simulink model "VehicleWithFourSpeedTransmission"  (R2025b)
settings: Solver=VariableStepAuto  StartTime=0.0  StopTime=50  FixedStep=1e-3  RelTol=1e-3  AbsTol=1e-3  EnableMultiTasking=on
model workspace (MAT data in the model file):
  DOWN_TABLE = [0  5  20  35; 0  5  20  35; 0  5  25  40; 0  5  30  50; 0  30  50  80; 0  30  50  80]
  DOWN_TH_BP = [0; 0.05; 0.4; 0.5; 0.9; 1]
  TWAIT = 2
  UP_TABLE = [10  30  50  1000000; 10  30  50  1000000; 15  30  50  1000000; 23  41  60  1000000; 40  70  100  1000000; 40  70  100  1000000]
  UP_TH_BP = [0; 0.25; 0.35; 0.5; 0.9; 1]
  clutchRise = 0.1
  eff_tor_rad = 0.4
  engagement_area = 0.0025
  fric_coeff = 0.5
  num_fric_surf = 6
  p0 = 2000000
  peak_normal = 0.55
  pressThresh = 0.05
  velTol = 0.001
libraries: sdl_lib x13, nesl_utility x12, fl_lib x11
CloseFcn:
  | try,close(h1_VehicleWithFourSpeedTransmission),end
  | clear h1_VehicleWithFourSpeedTransmission
  | 
  | clear simlog_VehicleWithFourSpeedTransmission
  | clear logsout_VehicleWithFourSpeedTransmission
Description:
  | Vehicle with Four-Speed Transmission
settings Model: FPTRunName=Active  ExtModeAutoUpdateStatusClock=off  Creator=The MathWorks, Inc.  LastModifiedBy=mateu
settings SolverCC: AutoScaleAbsTol=off  ZcThreshold=0  AlgebraicLoopSolver=TrustRegion
settings DataIOCC: LimitDataPoints=on  MaxDataPoints=10000  SaveOutput=off  DSMLogging=off  SaveTime=off  ReturnWorkspaceOutputs=off  SignalLoggingName=logsout_VehicleWithFourSpeedTransmission
settings OptimizationCC: ExpressionDepthLimit=2147483647.0  InitFltsAndDblsToZero=on  LifeSpan=inf
settings DebuggingCC: AlgebraicLoopMsg=none  SaveWithParameterizedLinksMsg=none  MergeDetectMultiDrivingBlocksExec=none  CheckExecutionContextPreStartOutputMsg=on  SignalResolutionControl=TryResolveAllWithWarning  MaskedZcDiagnostic=none  MultiTaskDSMMsg=warning  MultiTaskCondExecSysMsg=none  SigSpecEnsureSampleTimeMsg=none  UnconnectedInputMsg=warning  UnconnectedOutputMsg=warning  UnconnectedLineMsg=warning  AllowSymbolicDim=off  StateNameClashWarn=warning  PregeneratedLibrarySubsystemCodeDiagnostic=none  SFUnexpectedBacktrackingDiag=warning  SFNoUnconditionalDefaultTransitionDiag=warning  SFExecutionAtInitializationDiag=none  ArithmeticOperatorsInVariantConditions=warning
settings HardwareCC: ProdBitPerPointer=32.0  ProdBitPerSizeT=32.0  ProdBitPerPtrDiffT=32.0  ProdLargestAtomicFloat=None  ProdIntDivRoundTo=Undefined  ProdEndianess=Unspecified  ProdWordSize=32.0  ProdHWDeviceType=32-bit Generic  TargetBitPerPointer=64.0  TargetBitPerSizeT=64.0  TargetBitPerPtrDiffT=64.0  TargetLongLongMode=on  TargetIntDivRoundTo=Zero  TargetEndianess=LittleEndian  TargetWordSize=64.0  TargetHWDeviceType=MATLAB Host  ProdEqTarget=off
settings ModelReferenceCC: UpdateModelReferenceTargets=IfOutOfDate  EnableRefExpFcnMdlSchedulingChecks=on  PropagateSignalLabelsOutOfModel=off
settings SFSimCC: SimUseLocalCustomCode=off
settings RTWCC: RTWUseLocalCustomCode=off  GPUComputeCapability=3.5  DLArmComputeVersion=19.05
settings CodeAppCC: StateflowObjectComments=on
settings GRTTargetCC: TargetLangStandard=C89/C90 (ANSI)  CombineOutputUpdateFcns=off  GRTInterface=on
settings ConfigComp: CovScope=ReferencedModels  CovIncludeTopModel=off  CovMetricSettings=dw  CovSaveCumulativeToWorkspaceVar=on  CovSaveSingleToWorkspaceVar=on  CovExternalEMLEnable=off
settings SimscapeCC: SimscapeLogName=simlog_VehicleWithFourSpeedTransmission  SimscapeLogDataHistory=15000.0

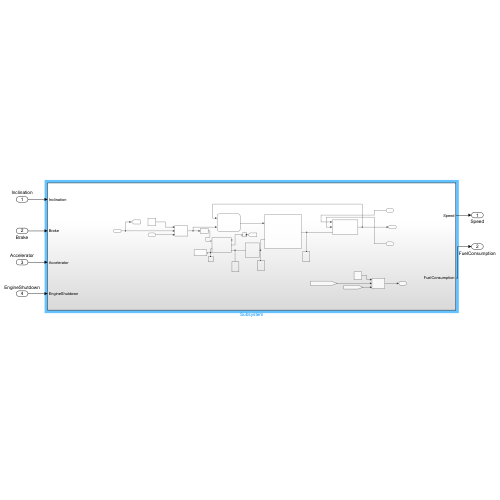
[thumbnail: Simulink's stored preview of the top-level diagram]
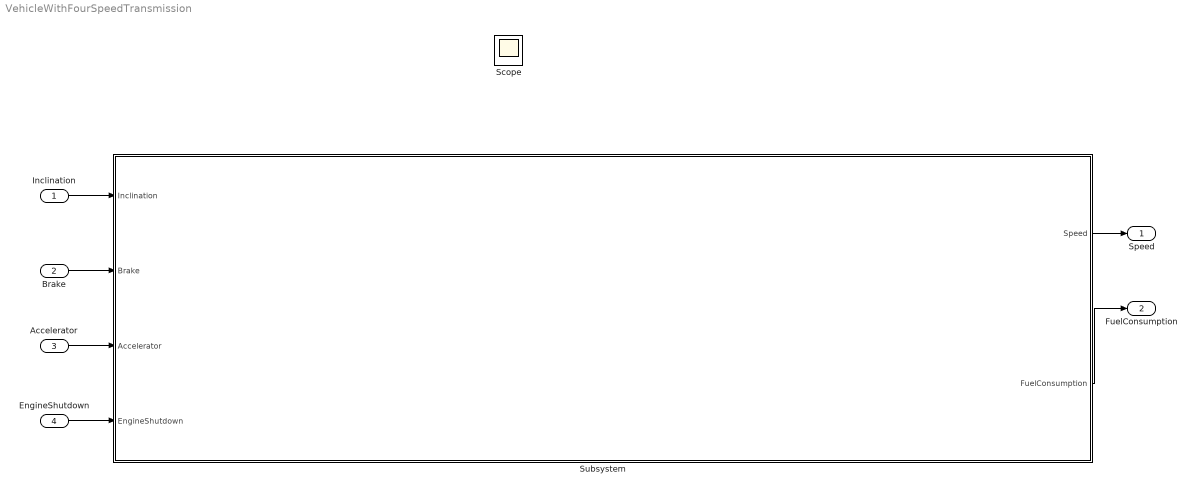
== system VehicleWithFourSpeedTransmission ==
  Inclination : Inport
  Brake : Inport  Port=2
  Accelerator : Inport  Port=3
  EngineShutdown : Inport  Port=4
  Subsystem : Subsystem
  Speed : Outport
  FuelConsumption : Outport  Port=2
  Scope : Scope
      settings: ActiveDisplayYMinimum=0.625  ActiveDisplayYMaximum=4.375
  wires:
  Inclination/1 -> Subsystem/1(Inclination)
  Brake/1 -> Subsystem/2(Brake)
  Accelerator/1 -> Subsystem/3(Accelerator)
  Subsystem/1(Speed) -> Speed/1
  Subsystem/2(FuelConsumption) -> FuelConsumption/1
  EngineShutdown/1 -> Subsystem/4(EngineShutdown)

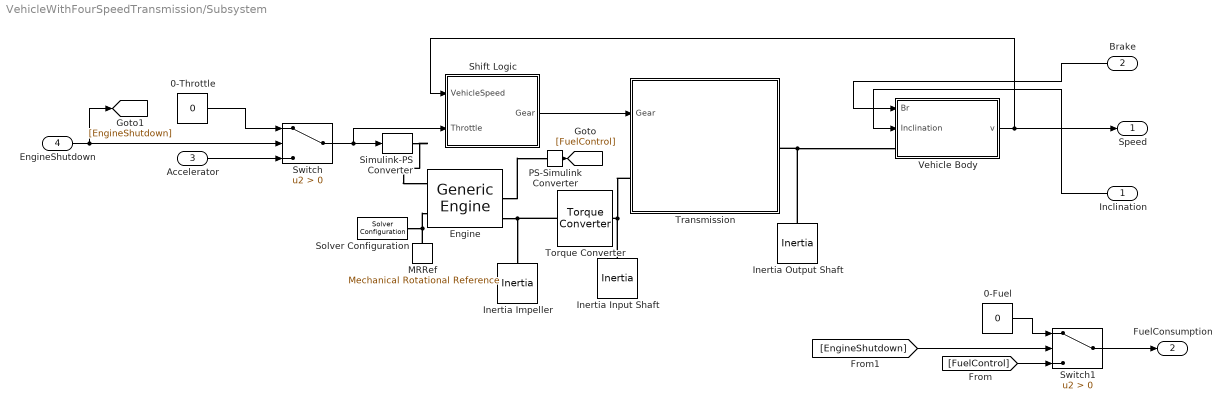
== system VehicleWithFourSpeedTransmission/Subsystem ==
  Inclination : Inport
  Brake : Inport  Port=2
  Accelerator : Inport  Port=3
  EngineShutdown : Inport  Port=4
  0-Fuel : Constant  Value=0
  0-Throttle : Constant  Value=0
  Engine : sdl_lib/Engines & Motors/Generic Engine  input_type=sdl.enum.GenericEngineInputType.NormalizedThrottle  model_parameterization=1  engine_type=1  Trq_max=380 N*m  w_Trq_max=4300 rpm  P_max=1.5e+5 W  w_P_max=4.5e+3 rpm  w_max=6e+3 rpm  w_min=500 rpm  w_tab=[ 500 1000 2e+3 3e+3 4e+3 5e+3 6e+3 7e+3 ] rpm  trq_tab=[ 380 380 380 380 350 280 200 80 ] N*m  pwr_tab=[ 2e+4 4e+4 7.8e+4 1.2e+5 1.45e+5 1.48e+5 1.25e+5 6e+4 ] W  interp_method=simscape.enum.interpolation.linear  w_thr=100 rpm  model_inertia=1  inertia=0.08 kg*m^2  initial_velocity=960 rpm  model_time_constant=1  time_constant=0.4 s  initial_normalized_throttle=0  fc_model=sdl.enum.fuel_consumption_model.FuelSpeedTorque  fc_per_rev=25 mg/rev  fc_w_tab=[ 1000 2e+3 3e+3 4e+3 5e+3 6e+3 ] rpm  fc_trq_tab=[ 0 80 160 200 240 320 360 400 ] N*m  fc_tab=[ 0.5 0.9 1.4 1.6 1.9 2.7 3.4 4.4; 1 1.7 2.7 3.1 3.6 5 6 7.4; 1.4 2.7 4 4.8 5.6 7.5 8.5 10.5; 2 3.6 5.8 6.7 8 10.4 11.7 13.3; 2.5 4.8 7.9 9.4 10.8 14 16.2 18.6; 3.1 6 10.3 11.9 13.8 18.4 22 26.5 ] g/s  bmep_tab=[ 0 250 500 625 750 1000 1.15e+3 1.25e+3 ] kPa  bsfc_tab=[ 410 380 300 280 270 290 320 380; 410 370 290 270 260 270 285 320; 415 380 290 275 265 270 270 300; 420 390 310 290 285 280 280 285; 430 410 340 320 310 300 310 320; 450 430 370 340 330 330 350 380 ] g/hr/kW  fc_interp_method=simscape.enum.interpolation.linear  displaced_volume=400 cm^3  rev_per_cycle=2  idle_speed=true  idle_speed_reference=1000 rpm  tau_controller=1 s  idle_w_thr=1 rpm  redline=0  redline_speed=5000 rpm  tau_redline=1 s  redline_w_thr=1 rpm
      settings: InternalSimscapePortConfiguration="{\"Bottom\":[],\"Left\":[{\"id\":\"ThrNorm\",\"label\":\"Thr\",\"type\":\"input\"},{\"id\":\"B\",\"label\":\"B\",\"type\":\"foundation.mechanical.rotational.rotational\"}],\"Right\":[{\"id\":\"P\",\"label\":\"P\",\"type\":\"output\"},{\"id\":\"FC\",\"label\":\"FC\",\"type\":\"output\"},{\"id\":\"F\",\"label\":\"F\",\"type\":\"foundation.mechanical.rotational.rotational\"}],\"Top\":[]}"
  Inertia Impeller : fl_lib/Mechanical/Rotational Elements/Inertia  inertia=0.02 kg*m^2  num_ports=foundation.enum.numPorts2.one  w_specify=on  w_priority=None  w=0 rpm  w_nominal_specify=off  w_nominal_value=1  w_nominal_unit=rad/s  t_specify=off  t_priority=High  t=0 N*m  t_nominal_specify=off  t_nominal_value=1  t_nominal_unit=N*m
  Inertia Input Shaft : fl_lib/Mechanical/Rotational Elements/Inertia  inertia=1e-2 kg*m^2  num_ports=foundation.enum.numPorts2.one  w_specify=on  w_priority=High  w=0 rad/s  w_nominal_specify=off  w_nominal_value=1  w_nominal_unit=rad/s  t_specify=off  t_priority=High  t=0 N*m  t_nominal_specify=off  t_nominal_value=1  t_nominal_unit=N*m
  Inertia Output Shaft : fl_lib/Mechanical/Rotational Elements/Inertia  inertia=1e-1 kg*m^2  num_ports=foundation.enum.numPorts2.one  w_specify=on  w_priority=None  w=0 rad/s  w_nominal_specify=off  w_nominal_value=1  w_nominal_unit=rad/s  t_specify=off  t_priority=High  t=0 N*m  t_nominal_specify=off  t_nominal_value=1  t_nominal_unit=N*m
  MRRef : fl_lib/Mechanical/Rotational Elements/Mechanical Rotational Reference
  PS-Simulink Converter : nesl_utility/PS-Simulink Converter  PhysicalDomain=network_engine_domain  SubClassName=ps_output  LeftPortType=input  RightPortType=output  PseudoPeriodic=off  Frequencies=[]  VectorFormat=inherit  Unit=inherit  AffineConversion=off
  Shift Logic : Stateflow chart  Tag=PublishSubsystem  TreatAsAtomicUnit=on
  Simulink-PS Converter : nesl_utility/Simulink-PS Converter  PhysicalDomain=network_engine_domain  SubClassName=ps_input  LeftPortType=input  RightPortType=output  PseudoPeriodic=off  Frequencies=[]  NoiseDistribution=none  NoiseParameters=[]  Unit=1  AffineConversion=off  FilteringAndDerivatives=zero  SimscapeFilterOrder=1  InputFilterTimeConstant=0.001  UdotUserProvided=1
  Solver Configuration : nesl_utility/Solver Configuration  PhysicalDomain=network_engine_domain  SubClassName=solver  LeftPortType=input  RightPortType=generic  Tones=[]  Harmonics=[]  SimulateNoise=off  Profile=off  UseLocalSampling=off  EnableSwitchedLinearOptims=on  FrequencyDomain=off  UseCCode=off  RelTol=0.001  AbsTol=1e-06  MinStep=1e-09  ToWorkspace=off  RevertToSquareIcSolve=off  NumHomotopyIterations=100  PhasorMode=off  PhasorModeNumHarmonics=1  ConsistencySolver=NEWTON_XTOL_AFTER_FTOL  IndexReductionMethod=DerivativeReplacement  DoDC=off  ResidualTolerance=1e-9  ConsistencyTolSource=GLOBAL  ConsistencyAbsTol=0.001  ConsistencyRelTol=0.001  ConsistencyTolFactor=0.001  UseLocalSolver=off  LocalSolverChoice=NE_PARTITIONING_ADVANCER  ResolveIndetEquations=on  FunctionEvalNumThread=1  LocalSolverSampleTime=0.005  DoFixedCost=off  MaxNonlinIter=6  MaxModeIter=2  ComputeImpulses=off  ImpulseIterations=2  LinearAlgebra=auto  LinearAlgebraNumThread=0  EquationFormulation=NE_TIME_EF  DelaysMemoryBudget=1024  AutomaticFiltering=on  FilteringTimeConstant=0.001  PartitionStorageMethod=EXHAUSTIVE  PartitionMemoryBudget=1024  PartitionMethod=ROBUST  MultibodyUseLocalSolver=off  MultibodyLocalSolverChoice=ODE1  MultibodyLocalSolverSampleTime=0.001
  Switch : Switch  Criteria=u2 > Threshold  SaturateOnIntegerOverflow=off  InputSameDT=off
  Switch1 : Switch  Criteria=u2 > Threshold  SaturateOnIntegerOverflow=off  InputSameDT=off
  Torque Converter : sdl_lib/Couplings & Drives/Torque Converter  coast_mode_modeling=sdl.enum.torqueConverterContinuousTwomode.continuous  SR_drive_tlu=[0, .5, .6, .7, .8, .87, .92, .94, .96, .97, 1]  TR_drive_tlu=[2.232, 1.5462, 1.4058, 1.2746, 1.1528, 1.0732, 1.0192, 1, 1, 1, 1]  CF_drive_tlu=1e-4 * [.72558, .66322, .63463, .59042, .51331, .4144, .29287, .22444, .12186, .04386, 0] m*N/rpm^2  SR_coast_tlu=[0, .5, .6, .7, .8, .87, .92, .94, .96, .97, 1]  CF_coast_tlu=1e-4 * [.5079, .4643, .4442, .4133, .3593, .2901, .205, .1571, .0853, .0307, 0] m*N/rpm^2  iniMode=sdl.enum.torqueConverterInitialMode.drive  delta_w=1 rpm  n_vector=[0 0.50 0.60 0.70 0.80 0.87 0.92 0.94 0.96 0.97]  trq_vector=[2.2320 1.5462 1.4058 1.2746 1.1528 1.0732 1.0192 0.9983 0.9983 0.9983]  cf_vector_parameterization=1  cf_vector_reference_speed=1  cf_vector=[12.2938 12.8588 13.1452 13.6285 14.6163 16.2675 19.3503 22.1046 29.9986 50.00] (rad/s)/(N*m)^0.5  cf_vector_sq=1e-3*[ 6.616 6.048 5.787 5.384 4.681 3.779 2.671 2.047 1.111 0.400] N*m/(rad/s)^2  interp_method=1  extrap_method=1  model_lag=0  tau=0.02 s  initial_trq_ratio=0
      settings: InternalSimscapePortConfiguration="{\"Bottom\":[],\"Left\":[{\"id\":\"I\",\"label\":\"I\",\"type\":\"foundation.mechanical.rotational.rotational\"}],\"Right\":[{\"id\":\"T\",\"label\":\"T\",\"type\":\"foundation.mechanical.rotational.rotational\"}],\"Top\":[]}"
  Transmission : Subsystem  Tag=PublishSubsystem
      mask Display:
      | % Icon data
      | Icon.x1 = [-1.3 -1.1 -1.1 -1 -1 -1 -0.9 -0.9 -0.9 -0.8 -0.8];
      | Icon.x1_1 = [-0.8 -0.7 -0.7 -0.7 -0.6 -0.6 -0.6 -0.5 -0.5 -0.5];
      | Icon.y1 = [0 0 0.15 0.15 0.05 0.15 0.15 0.05 0.15 0.15 0.05];
      | Icon.y1_1 =[0.15 0.15 0.05 0.15 0.15 0.07 0.15 0.15 0.07 0.15];
      | Icon.x2 = [-1.05 -1.05 -0.95 -0.95 -0.95 0.3];
      | Icon.y2 = [0.08   0     0     0.08  0    0];
      | Icon.x3 = [-0.85 -0.85 -0.75 -0.75 -0.75 0 0 -0.3 -0.3  0.3];
      | Icon.y3 = [0.08 0.02 0.02 0.08 0.02 0.02 0.15 0.15 0.33 0.33];
      | Icon.x3_1 = [-0.65 -0.65 -0.55 -0.55 -0.55 -0.4];
      | Icon.y3_1 = [0.1    0.05  0.05  0.1   0.05 0.05];
      | Icon.x4 = [-0.2 -0.1 -0.15 -0.15 -0.2 -0.1];
      | Icon.y4 = [0.12 0.12 0.12 0.18 0.18 0.18];
      | Icon.x5 = [-0.2 -0.1 -0.1 -0.15 -0.15 -0.4 -0.4];
      | Icon.y5 = [0.1 0.1 0.1 0.1 0.05 0.05 0.4];
      | Icon.x6 = [-0.2 -0.1 -0.15 -0.15 0.1 0.1 0.4 0.4];
      | Icon.y6 = [0.20 0.20 0.20 0.3 0.3 0.19 0.19 0];
      | Icon.x7 = [0.3 0.3 0.25 0.35];
      | Icon.y7 = [0 0.13 0.13 0.13];
      | Icon.x8 = [0.25 0.35 0.3 0.3 0.25 0.35];
      | Icon.y8 = [0.15 0.15 0.15 0.23 0.23 0.23];
      | Icon.x9 = [0.25 0.35 0.3 0.3];
      | Icon.y9 = [0.25 0.25 0.25 0.40];
      | Icon.x10 = [0.25 0.25 0.35 0.35 0.35 0.15 0.15 0.15];
      | Icon.y10 = [0.35 0.45 0.45 0.35 0.45 0.45 0.35 0.45];
      | Icon.x11 = [0.2 0.2];
      | Icon.y11 = [0.33 0.40];
      | Icon.x12 = [0.4 0.6];
      | Icon.y12 = [0 0];
      | Icon.x13 = [-0.45 -0.45 -0.35 -0.35 -0.35 -0.55 -0.55];
      | Icon.y13 = [0.35 0.45 0.45 0.35 0.45 0.45 0.35];
      | Icon.x14 = [-0.4 -0.5 -0.5];
      | Icon.y14 = [0.33 0.33 0.4];
      | Icon.x15 = [-0.5 0.35];
      | Icon.y15 = [0.45 0.45];
      | Icon.x16 = [-1.3 -1.1 -1.1 -1 -1 -1 -0.9 -0.9 ];
      | Icon.x16_1 = [-0.9 -0.8 -0.8 -0.8 -0.7 -0.7 -0.7 -0.6];
      | Icon.x16_2 = [-0.6 -0.6 -0.5 -0.5 -0.5];
      | Icon.y16 = [0 0 -0.15 -0.15 -0.05 -0.15 -0.15 -0.05];
      | Icon.y16_1 = [-0.15 -0.15 -0.05 -0.15 -0.15 -0.05 -0.15 -0.15];
      | Icon.y16_2 = [-0.07 -0.15 -0.15 -0.07 -0.15];
      | Icon.x17 = [-1.05 -1.05 -0.95 -0.95 -0.95 0.3];
      | Icon.y17 = [-0.08 0 0 -0.08 0 0];
      | Icon.x18 = [-0.85 -0.85 -0.75 -0.75 -0.75 0 0 -0.3];
      | Icon.x18_1 = [-0.3  0.3];
      | Icon.x18_2 = [-0.65 -0.65 -0.55 -0.55 -0.55 -0.4];
      | Icon.y18 = [-0.08 -0.02 -0.02 -0.08 -0.02 -0.02 -0.15 -0.15];
      | Icon.y18_1 = [-0.33 -0.33];
      | Icon.y18_2 = [-0.1 -0.05 -0.05 -0.1 -0.05 -0.05];
      | Icon.x19 = [-0.2 -0.1 -0.15 -0.15 -0.2 -0.1];
      | Icon.y19 = [-0.12 -0.12 -0.12 -0.18 -0.18 -0.18];
      | Icon.x20 = [-0.2 -0.1 -0.1 -0.15 -0.15 -0.4 -0.4];
      | Icon.y20 = [-0.1 -0.1 -0.1 -0.1 -0.05 -0.05 -0.4];
      | Icon.x21 = [-0.2 -0.1 -0.15 -0.15 0.1 0.1 0.4 0.4];
      | Icon.y21 = [-0.20 -0.20 -0.20 -0.3 -0.3 -0.19 -0.19 0];
      | Icon.x22 = [0.3 0.3 0.25 0.35];
      | Icon.y22 = [0 -0.13 -0.13 -0.13];
      | Icon.x23 = [0.25 0.35 0.3 0.3 0.25 0.35];
      | Icon.y23 = [-0.15 -0.15 -0.15 -0.23 -0.23 -0.23];
      | Icon.x24 = [0.25 0.35 0.3 0.3];
      | Icon.y24 = [-0.25 -0.25 -0.25 -0.40];
      | Icon.x25 = [0.25 0.25 0.35 0.35 0.35 0.15 0.15 0.15];
      | Icon.y25 = [-0.35 -0.45 -0.45 -0.35 -0.45 -0.45 -0.35 -0.45];
      | Icon.x26 = [0.2 0.2];
      | Icon.y26 = [-0.33 -0.40];
      | Icon.x27 = [-0.45 -0.45 -0.35 -0.35 -0.35 -0.55 -0.55];
      | Icon.y27 = [-0.35 -0.45 -0.45 -0.35 -0.45 -0.45 -0.35];
      | Icon.x28 = [-0.4 -0.5 -0.5];
      | Icon.y28 = [-0.33 -0.33 -0.4];
      | Icon.x29 = [-0.5 0.35];
      | Icon.y29 = [-0.45 -0.45];
      | % Bounding box
      | Icon.LowerLeftx = -1.4;
      | Icon.LowerLefty = -0.55;
      | Icon.UpperRightx = 1.0;
      | Icon.UpperRighty = 0.55;
      | 
      | plot(Icon.x1,Icon.y1);
      | plot(Icon.x1_1,Icon.y1_1);
      | plot(Icon.x2,Icon.y2);
      | plot(Icon.x3,Icon.y3);
      | plot(Icon.x3_1,Icon.y3_1);
      | plot(Icon.x4,Icon.y4);
      | plot(Icon.x5,Icon.y5);
      | plot(Icon.x6,Icon.y6);
      | plot(Icon.x7,Icon.y7);
      | plot(Icon.x8,Icon.y8);
      | plot(Icon.x9,Icon.y9);
      | plot(Icon.x10,Icon.y10);
      | plot(Icon.x11,Icon.y11);
      | plot(Icon.x12,Icon.y12);
      | plot(Icon.x13,Icon.y13);
      | plot(Icon.x14,Icon.y14);
      | plot(Icon.x15,Icon.y15);
      | plot(Icon.x16,Icon.y16);
      | plot(Icon.x16_1,Icon.y16_1);
      | plot(Icon.x16_2,Icon.y16_2);
      | plot(Icon.x17,Icon.y17);
      | plot(Icon.x18,Icon.y18);
      | plot(Icon.x18_1,Icon.y18_1);
      | plot(Icon.x18_2,Icon.y18_2);
      | plot(Icon.x19,Icon.y19);
      | plot(Icon.x20,Icon.y20);
      | plot(Icon.x21,Icon.y21);
      | plot(Icon.x22,Icon.y22);
      | plot(Icon.x23,Icon.y23);
      | plot(Icon.x24,Icon.y24);
      | plot(Icon.x25,Icon.y25);
      | plot(Icon.x26,Icon.y26);
      | plot(Icon.x27,Icon.y27);
      | plot(Icon.x28,Icon.y28);
      | plot(Icon.x29,Icon.y29);
      | 
      | plot(Icon.LowerLeftx,Icon.LowerLefty);
      | plot(Icon.UpperRightx,Icon.UpperRighty);
  Vehicle Body : Subsystem  Tag=PublishSubsystem
      mask Display:
      | color('white')
      | plot(-120,-60); plot(120,50);
      | color('black')
      | plot(sin(0:0.1:6*pi)*15-70,cos(0:0.1:6*pi)*15-30);
      | plot(sin(0:0.1:6*pi)*15+70,cos(0:0.1:6*pi)*15-30);
      | plot([-88 -95 -99 -99 -95 -75 -65 -50 -46 10 30 34 80 85 90 93 95 93 90 88],[-30 -28 -23 -5 0 5 10 20 21 21 0 -2 -7 -9 -13 -17 -25 -28 -30 -30])
      | plot([-88 -95 -99 -99 -95 -75 -65 -50 -46 10 30 34 80 85 90 93 95 93 90 88],[-30 -28 -23 -5 0 5 10 20 21 21 0 -2 -7 -9 -13 -17 -25 -28 -30 -30]-1)
      | plot([-88 -95 -99 -99 -95 -75 -65 -50 -46 10 30 34 80 85 90 93 95 93 90 88]+1,[-30 -28 -23 -5 0 5 10 20 21 21 0 -2 -7 -9 -13 -17 -25 -28 -30 -30])
      | plot([-50 50],[-30 -30])
  Speed : Outport
  FuelConsumption : Outport  Port=2
  wires:
  Shift Logic/1(Gear) -> Transmission/1(Gear)
  Vehicle Body/1(v) -> Speed/1, Shift Logic/1(VehicleSpeed)
  Brake/1 -> Vehicle Body/1(Br)
  Inclination/1 -> Vehicle Body/2(Inclination)
  Switch/1 -> Shift Logic/2(Throttle), Simulink-PS Converter/1
  Accelerator/1 -> Switch/3
  EngineShutdown/1 -> [EngineShutdown], Switch/2
  0-Throttle/1 -> Switch/1
  PS-Simulink Converter/1 -> [FuelControl]
  [EngineShutdown] -> Switch1/2
  0-Fuel/1 -> Switch1/1
  [FuelControl] -> Switch1/3
  Switch1/1 -> FuelConsumption/1
  connections:
  Simulink-PS Converter/RConn1 -- Engine/LConn1
  Engine/RConn2 -- PS-Simulink Converter/LConn1
  MRRef/LConn1 -- Solver Configuration/RConn1 -- Engine/LConn2
  Torque Converter/LConn1 -- Inertia Impeller/LConn1 -- Engine/RConn3
  Transmission/LConn1 -- Torque Converter/RConn1 -- Inertia Input Shaft/LConn1
  Inertia Output Shaft/LConn1 -- Transmission/RConn1 -- Vehicle Body/LConn1

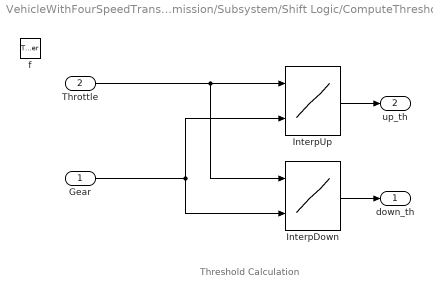
== system VehicleWithFourSpeedTransmission/Subsystem/Shift Logic/ComputeThreshold ==
  note: Threshold Calculation
  Gear : Inport
  Throttle : Inport  Port=2
  f : TriggerPort  TriggerType=function-call  VariantControl=Variant
      settings: CopyFcn=Stateflow.SLINSF.SimulinkMan.removeBlockPreDeleteFcn  PreDeleteFcn=Stateflow.SLINSF.SimulinkMan.unsafePredeleteFcn
  InterpDown : Lookup_n-D  LookupTableObject=''  BreakpointsForDimension1=DOWN_TH_BP  BreakpointsForDimension2=[1:4]  Table=DOWN_TABLE  OutDataTypeStr=double  InputSameDT=off  LockScale=on
      settings: InputPortMap=u0,u1
  InterpUp : Lookup_n-D  LookupTableObject=''  BreakpointsForDimension1=UP_TH_BP  BreakpointsForDimension2=[1:4]  Table=UP_TABLE  OutDataTypeStr=double  InputSameDT=off  LockScale=on
      settings: InputPortMap=u0,u1
  down_th : Outport  InitialOutput=0  VectorParamsAs1DForOutWhenUnconnected=off
  up_th : Outport  Port=2  InitialOutput=0  VectorParamsAs1DForOutWhenUnconnected=off
  wires:
  InterpUp/1 -> up_th/1
  InterpDown/1 -> down_th/1
  Throttle/1 -> InterpDown/1, InterpUp/1
  Gear/1 -> InterpDown/2, InterpUp/2

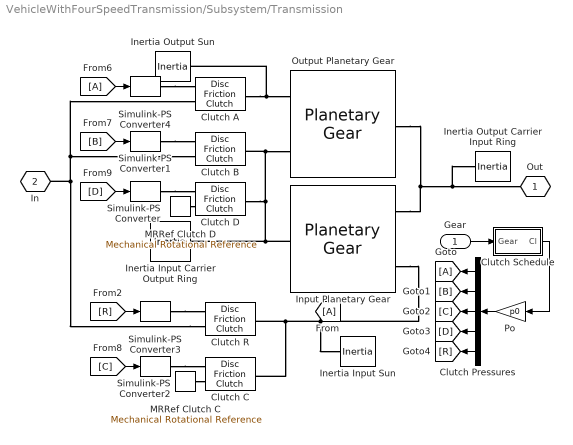
== system VehicleWithFourSpeedTransmission/Subsystem/Transmission ==
  Gear : Inport
  Clutch Pressures : Demux  Outputs=5
  Clutch Schedule : Subsystem  Tag=PublishSubsystem
  Clutch A : sdl_lib/Clutches/Disc Friction Clutch  geometry_model=1  r_eff=eff_tor_rad m  d_o=0.15 m  d_i=0.1 m  nS=num_fric_surf  piston_area=engagement_area m^2  unidirectional=0  friction_model=1  mu_w_vector=[ 0 0.1 0.2 0.3 0.4 0.5 1 2 5 10 100 1000 ] rad/s  temperature_TLU=[280.0, 300.0, 320.0] K  mu_static=peak_normal  mu_static_vector=[0.4, 0.38, 0.36]  mu_coulomb=fric_coeff  mu_coulomb_vector=[ 0.29 0.28 0.26 0.22 0.21 0.2 0.2 0.19 0.19 0.19 0.19 0.19 ]  mu_coulomb_temp_vector=[0.3, 0.28, 0.25]  mu_coulomb_matrix=[0.34, 0.32, 0.3; 0.3, 0.28, 0.25; 0.25, 0.2, 0.15]  mu_interp_method=simscape.enum.interpolation.linear  mu_extrap_method=simscape.enum.extrapolation.linear  d_f=1  w_tol=velTol rad/s  pressure_min=pressThresh*p0 Pa  mu_visc=0 N*m/(rad/s)  initial_state_locked=0  thermal_mass=25 kJ/K  T_init=300 K
      settings: InternalSimscapePortConfiguration="{\"Bottom\":[],\"Left\":[{\"id\":\"P\",\"label\":\"P\",\"type\":\"input\"},{\"id\":\"B\",\"label\":\"B\",\"type\":\"foundation.mechanical.rotational.rotational\"}],\"Right\":[{\"id\":\"F\",\"label\":\"F\",\"type\":\"foundation.mechanical.rotational.rotational\"}],\"Top\":[]}"
  Clutch B : sdl_lib/Clutches/Disc Friction Clutch  geometry_model=1  r_eff=eff_tor_rad m  d_o=0.15 m  d_i=0.1 m  nS=num_fric_surf  piston_area=engagement_area m^2  unidirectional=0  friction_model=1  mu_w_vector=[ 0 0.1 0.2 0.3 0.4 0.5 1 2 5 10 100 1000 ] rad/s  temperature_TLU=[280.0, 300.0, 320.0] K  mu_static=peak_normal  mu_static_vector=[0.4, 0.38, 0.36]  mu_coulomb=fric_coeff  mu_coulomb_vector=[ 0.29 0.28 0.26 0.22 0.21 0.2 0.2 0.19 0.19 0.19 0.19 0.19 ]  mu_coulomb_temp_vector=[0.3, 0.28, 0.25]  mu_coulomb_matrix=[0.34, 0.32, 0.3; 0.3, 0.28, 0.25; 0.25, 0.2, 0.15]  mu_interp_method=1  mu_extrap_method=1  d_f=1  w_tol=velTol rad/s  pressure_min=pressThresh*p0 Pa  mu_visc=0 N*m/(rad/s)  initial_state_locked=0  thermal_mass=25 kJ/K  T_init=300 K
      settings: InternalSimscapePortConfiguration="{\"Bottom\":[],\"Left\":[{\"id\":\"P\",\"label\":\"P\",\"type\":\"input\"},{\"id\":\"B\",\"label\":\"B\",\"type\":\"foundation.mechanical.rotational.rotational\"}],\"Right\":[{\"id\":\"F\",\"label\":\"F\",\"type\":\"foundation.mechanical.rotational.rotational\"}],\"Top\":[]}"
  Clutch C : sdl_lib/Clutches/Disc Friction Clutch  geometry_model=1  r_eff=eff_tor_rad m  d_o=0.15 m  d_i=0.1 m  nS=num_fric_surf  piston_area=engagement_area m^2  unidirectional=0  friction_model=1  mu_w_vector=[ 0 0.1 0.2 0.3 0.4 0.5 1 2 5 10 100 1000 ] rad/s  temperature_TLU=[280.0, 300.0, 320.0] K  mu_static=peak_normal  mu_static_vector=[0.4, 0.38, 0.36]  mu_coulomb=fric_coeff  mu_coulomb_vector=[ 0.29 0.28 0.26 0.22 0.21 0.2 0.2 0.19 0.19 0.19 0.19 0.19 ]  mu_coulomb_temp_vector=[0.3, 0.28, 0.25]  mu_coulomb_matrix=[0.34, 0.32, 0.3; 0.3, 0.28, 0.25; 0.25, 0.2, 0.15]  mu_interp_method=1  mu_extrap_method=1  d_f=1  w_tol=velTol rad/s  pressure_min=pressThresh*p0 Pa  mu_visc=0 N*m/(rad/s)  initial_state_locked=0  thermal_mass=25 kJ/K  T_init=300 K
      settings: InternalSimscapePortConfiguration="{\"Bottom\":[],\"Left\":[{\"id\":\"P\",\"label\":\"P\",\"type\":\"input\"},{\"id\":\"B\",\"label\":\"B\",\"type\":\"foundation.mechanical.rotational.rotational\"}],\"Right\":[{\"id\":\"F\",\"label\":\"F\",\"type\":\"foundation.mechanical.rotational.rotational\"}],\"Top\":[]}"
  Clutch D : sdl_lib/Clutches/Disc Friction Clutch  geometry_model=1  r_eff=eff_tor_rad m  d_o=0.15 m  d_i=0.1 m  nS=num_fric_surf  piston_area=engagement_area m^2  unidirectional=0  friction_model=1  mu_w_vector=[ 0 0.1 0.2 0.3 0.4 0.5 1 2 5 10 100 1000 ] rad/s  temperature_TLU=[280.0, 300.0, 320.0] K  mu_static=peak_normal  mu_static_vector=[0.4, 0.38, 0.36]  mu_coulomb=fric_coeff  mu_coulomb_vector=[ 0.29 0.28 0.26 0.22 0.21 0.2 0.2 0.19 0.19 0.19 0.19 0.19 ]  mu_coulomb_temp_vector=[0.3, 0.28, 0.25]  mu_coulomb_matrix=[0.34, 0.32, 0.3; 0.3, 0.28, 0.25; 0.25, 0.2, 0.15]  mu_interp_method=simscape.enum.interpolation.linear  mu_extrap_method=simscape.enum.extrapolation.linear  d_f=1  w_tol=velTol rad/s  pressure_min=pressThresh*p0 Pa  mu_visc=0 N*m/(rad/s)  initial_state_locked=0  thermal_mass=25 kJ/K  T_init=300 K
      settings: InternalSimscapePortConfiguration="{\"Bottom\":[],\"Left\":[{\"id\":\"P\",\"label\":\"P\",\"type\":\"input\"},{\"id\":\"B\",\"label\":\"B\",\"type\":\"foundation.mechanical.rotational.rotational\"}],\"Right\":[{\"id\":\"F\",\"label\":\"F\",\"type\":\"foundation.mechanical.rotational.rotational\"}],\"Top\":[]}"
  Clutch R : sdl_lib/Clutches/Disc Friction Clutch  geometry_model=1  r_eff=eff_tor_rad m  d_o=0.15 m  d_i=0.1 m  nS=num_fric_surf  piston_area=engagement_area m^2  unidirectional=0  friction_model=1  mu_w_vector=[ 0 0.1 0.2 0.3 0.4 0.5 1 2 5 10 100 1000 ] rad/s  temperature_TLU=[280.0, 300.0, 320.0] K  mu_static=peak_normal  mu_static_vector=[0.4, 0.38, 0.36]  mu_coulomb=fric_coeff  mu_coulomb_vector=[ 0.29 0.28 0.26 0.22 0.21 0.2 0.2 0.19 0.19 0.19 0.19 0.19 ]  mu_coulomb_temp_vector=[0.3, 0.28, 0.25]  mu_coulomb_matrix=[0.34, 0.32, 0.3; 0.3, 0.28, 0.25; 0.25, 0.2, 0.15]  mu_interp_method=1  mu_extrap_method=1  d_f=1  w_tol=velTol rad/s  pressure_min=pressThresh*p0 Pa  mu_visc=0 N*m/(rad/s)  initial_state_locked=0  thermal_mass=25 kJ/K  T_init=300 K
      settings: InternalSimscapePortConfiguration="{\"Bottom\":[],\"Left\":[{\"id\":\"P\",\"label\":\"P\",\"type\":\"input\"},{\"id\":\"B\",\"label\":\"B\",\"type\":\"foundation.mechanical.rotational.rotational\"}],\"Right\":[{\"id\":\"F\",\"label\":\"F\",\"type\":\"foundation.mechanical.rotational.rotational\"}],\"Top\":[]}"
  From : From
  From6 : From
  Goto : Goto
  Inertia Input Sun : fl_lib/Mechanical/Rotational Elements/Inertia  inertia=1e-4 kg*m^2  num_ports=foundation.enum.numPorts2.one  w_specify=on  w_priority=None  w=0 rad/s  w_nominal_specify=off  w_nominal_value=1  w_nominal_unit=rad/s  t_specify=off  t_priority=High  t=0 N*m  t_nominal_specify=off  t_nominal_value=1  t_nominal_unit=N*m
  Inertia Input Carrier Output Ring : fl_lib/Mechanical/Rotational Elements/Inertia  inertia=1e-4 kg*m^2  num_ports=foundation.enum.numPorts2.one  w_specify=on  w_priority=None  w=0 rad/s  w_nominal_specify=off  w_nominal_value=1  w_nominal_unit=rad/s  t_specify=off  t_priority=High  t=0 N*m  t_nominal_specify=off  t_nominal_value=1  t_nominal_unit=N*m
  Inertia Output Carrier Input Ring : fl_lib/Mechanical/Rotational Elements/Inertia  inertia=1e-4 kg*m^2  num_ports=foundation.enum.numPorts2.one  w_specify=on  w_priority=None  w=0 rad/s  w_nominal_specify=off  w_nominal_value=1  w_nominal_unit=rad/s  t_specify=off  t_priority=High  t=0 N*m  t_nominal_specify=off  t_nominal_value=1  t_nominal_unit=N*m
  Inertia Output Sun : fl_lib/Mechanical/Rotational Elements/Inertia  inertia=1e-4 kg*m^2  num_ports=foundation.enum.numPorts2.one  w_specify=on  w_priority=None  w=0 rad/s  w_nominal_specify=off  w_nominal_value=1  w_nominal_unit=rad/s  t_specify=off  t_priority=High  t=0 N*m  t_nominal_specify=off  t_nominal_value=1  t_nominal_unit=N*m
  "Input Planetary Gear " : sdl_lib/Gears/Planetary Gear  rs_ratio=2.2258  friction_model=1  efficiency=[ 0.96 0.98 ]  temperature_TLU=[ 280 300 320 ] K  efficiency_sp_TLU=[ 0.95 0.9 0.85 ]  efficiency_rp_TLU=[ 0.95 0.9 0.85 ]  pwr_thr=[ 0.001 0.001 ] W  mu_visc=[ 0 0 ] N*m/(rad/s)  model_inertia=0  sun_inertia=1e-10 kg*m^2  ring_inertia=1e-10 kg*m^2  carrier_inertia=1e-10 kg*m^2  carrier_radius=0.01 m  planet_inertia=0.001 kg*m^2  planet_mass=1e-10 kg  thermal_mass=50 J/K  T_init=300 K
  MRRef Clutch C : fl_lib/Mechanical/Rotational Elements/Mechanical Rotational Reference
  MRRef Clutch D : fl_lib/Mechanical/Rotational Elements/Mechanical Rotational Reference
  Output Planetary Gear : sdl_lib/Gears/Planetary Gear  rs_ratio=1.84  friction_model=1  efficiency=[ 0.96 0.98 ]  temperature_TLU=[ 280 300 320 ] K  efficiency_sp_TLU=[ 0.95 0.9 0.85 ]  efficiency_rp_TLU=[ 0.95 0.9 0.85 ]  pwr_thr=[ 0.001 0.001 ] W  mu_visc=[0 0] N*m/(rad/s)  model_inertia=0  sun_inertia=1e-10 kg*m^2  ring_inertia=1e-10 kg*m^2  carrier_inertia=1e-10 kg*m^2  carrier_radius=0.01 m  planet_inertia=0.001 kg*m^2  planet_mass=1e-10 kg  thermal_mass=50 J/K  T_init=300 K
  Po : Gain  Gain=p0
  Simulink-PS Converter{,1..4} (5 alike) : nesl_utility/Simulink-PS Converter  PhysicalDomain=network_engine_domain  SubClassName=ps_input  LeftPortType=input  RightPortType=output  PseudoPeriodic=off  Frequencies=[]  NoiseDistribution=none  NoiseParameters=[]  Unit=1  AffineConversion=off  FilteringAndDerivatives=zero  SimscapeFilterOrder=1  InputFilterTimeConstant=.001  UdotUserProvided=0
  Out : PMIOPort  Tag=PMCPort  Side=Right
  In : PMIOPort  Tag=PMCPort  Port=2  Side=Left
  wires:
  From6/1 -> Simulink-PS Converter4/1
  [R] -> Simulink-PS Converter3/1
  [C] -> Simulink-PS Converter2/1
  [B] -> Simulink-PS Converter1/1
  [D] -> Simulink-PS Converter/1
  Clutch Pressures/5 -> [R]
  Clutch Pressures/4 -> [D]
  Clutch Pressures/3 -> [C]
  Clutch Pressures/2 -> [B]
  Clutch Pressures/1 -> Goto/1
  Clutch Schedule/1(Cl) -> Po/1
  Po/1 -> Clutch Pressures/1
  Gear/1 -> Clutch Schedule/1(Gear)
  connections:
  Simulink-PS Converter4/RConn1 -- Clutch A/LConn1
  Simulink-PS Converter3/RConn1 -- Clutch R/LConn1
  Simulink-PS Converter2/RConn1 -- Clutch C/LConn1
  MRRef Clutch C/LConn1 -- Clutch C/LConn2
  Clutch R/LConn2 -- Clutch A/LConn2 -- Clutch B/LConn2 -- In/RConn1
  Simulink-PS Converter1/RConn1 -- Clutch B/LConn1
  "Input Planetary Gear "/LConn1 -- Inertia Input Carrier Output Ring/LConn1 -- Clutch D/RConn1 -- Clutch B/RConn1 -- Output Planetary Gear/RConn1
  Clutch C/RConn1 -- "Input Planetary Gear "/RConn2 -- Inertia Input Sun/LConn1 -- Clutch R/RConn1
  Simulink-PS Converter/RConn1 -- Clutch D/LConn1
  MRRef Clutch D/LConn1 -- Clutch D/LConn2
  Clutch A/RConn1 -- Output Planetary Gear/RConn2 -- Inertia Output Sun/LConn1
  Output Planetary Gear/LConn1 -- "Input Planetary Gear "/RConn1 -- Out/RConn1 -- Inertia Output Carrier Input Ring/LConn1

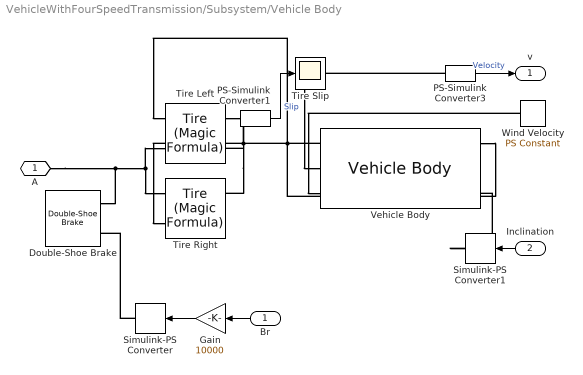
== system VehicleWithFourSpeedTransmission/Subsystem/Vehicle Body ==
  Br : Inport
  Inclination : Inport  Port=2
  Double-Shoe Brake : sdl_lib/Brakes & Detents/Rotational/Double-Shoe Brake  r_drum=150 mm  r_act=100 mm  r_pin=125 mm  theta_pin=15 deg  theta_0=5 deg  theta_shoe=120 deg  mu_visc=.01 N*m/(rad/s)  thermal_port=simscape.enum.thermaleffects.omit  mu=0.3  temperature_TLU=[280.0, 300.0, 320.0] K  mu_TLU=[0.1, 0.05, 0.03]  w_thr=0.01 rad/s  thermal_mass=50 kJ/K  temperature_specify=off  temperature_priority=High  temperature=300 K  temperature_nominal_specify=off  temperature_nominal_value=1  temperature_nominal_unit=K
      settings: InternalSimscapePortConfiguration="{\"Bottom\":[],\"Left\":[{\"id\":\"F\",\"label\":\"F\",\"type\":\"input\"},{\"id\":\"S\",\"label\":\"S\",\"type\":\"foundation.mechanical.rotational.rotational\"}],\"Right\":[],\"Top\":[]}"
  Gain : Gain  Gain=10000
  PS-Simulink Converter1 : nesl_utility/PS-Simulink Converter  PhysicalDomain=network_engine_domain  SubClassName=ps_output  LeftPortType=input  RightPortType=output  PseudoPeriodic=off  Frequencies=[]  VectorFormat=1-D array  Unit=1  AffineConversion=off
  PS-Simulink Converter3 : nesl_utility/PS-Simulink Converter  PhysicalDomain=network_engine_domain  SubClassName=ps_output  LeftPortType=input  RightPortType=output  PseudoPeriodic=off  Frequencies=[]  VectorFormat=1-D array  Unit=mph  AffineConversion=off
  Simulink-PS Converter : nesl_utility/Simulink-PS Converter  PhysicalDomain=network_engine_domain  SubClassName=ps_input  LeftPortType=input  RightPortType=output  PseudoPeriodic=off  Frequencies=[]  NoiseDistribution=none  NoiseParameters=[]  Unit=1  AffineConversion=off  FilteringAndDerivatives=zero  SimscapeFilterOrder=1  InputFilterTimeConstant=0.001  UdotUserProvided=1
  Simulink-PS Converter1 : nesl_utility/Simulink-PS Converter  PhysicalDomain=network_engine_domain  SubClassName=ps_input  LeftPortType=input  RightPortType=output  PseudoPeriodic=off  Frequencies=[]  NoiseDistribution=none  NoiseParameters=[]  Unit=1  AffineConversion=off  FilteringAndDerivatives=zero  SimscapeFilterOrder=1  InputFilterTimeConstant=0.001  UdotUserProvided=1
  Tire Slip : Scope
      settings: ActiveDisplayYMinimum=-1.12689  ActiveDisplayYMaximum=0.14199
  Tire Left : sdl_lib/Tires & Vehicles/Tire (Magic Formula)  parameterization=1  F_z1=3000 N  F_x1=3500 N  kappa1=10  B_m=10  C_m=1.9  D_m=1  E_m=0.97  fz0=4e+3 N  p_Cx=1.685  p_Dx=[ 1.21 -0.037 ]  p_Ex=[ 0.344 0.095 -0.02 0 ]  p_Kx=[ 21.51 -0.163 0.245 ]  p_Hx=[ -0.002 0.002 ]  p_Vx=[ 0 0 ]  rolling_radius_model=sdl.enum.RollingRadiusParameterization.Constant  r_e=0.3 m  r_0=0.3 m  breff=8.39  dreff=0.26  freff=0.074  q_re0=0.99  q_v1=0.008  longvl=17 m/s  cz=5e5 N/m  model_resistance=0  resistance_model=1  coeff=0.015  p_tire=250e3 Pa  alpha=-0.003  beta=0.97  coeff_a=84e-4  coeff_b=6.2e-4 s/m  coeff_c=1.6e-4 s^2/m^2  p_tire0=240e3 Pa  fz0_resistance=4000 N  vH0=16 m/s  q_Sy=[.0082, 0, .0014, .001, 0, 0, 1.08, -.5]  v_thr=1e-3 m/s  enable_scaling_coefficients=false  lfzO=1  lcx=1  lmux=1  lex=1  lkx=1  lhx=1  lvx=1  lmy=1  model_compliance=0  stiffness=1e+6 N/m  damping=1000 N/(m/s)  model_inertia=1  inertia=1e-2 kg*m^2  initial_velocity=0 rpm  vxlow=0.1 m/s  v_tr_thr=0.01 m/s  kpumin=-1.5  kpumax=1.5
  Tire Right : sdl_lib/Tires & Vehicles/Tire (Magic Formula)  parameterization=1  F_z1=3000 N  F_x1=3500 N  kappa1=10  B_m=10  C_m=1.9  D_m=1  E_m=0.97  fz0=4e+3 N  p_Cx=1.685  p_Dx=[ 1.21 -0.037 ]  p_Ex=[ 0.344 0.095 -0.02 0 ]  p_Kx=[ 21.51 -0.163 0.245 ]  p_Hx=[ -0.002 0.002 ]  p_Vx=[ 0 0 ]  rolling_radius_model=sdl.enum.RollingRadiusParameterization.Constant  r_e=0.3 m  r_0=0.3 m  breff=8.39  dreff=0.26  freff=0.074  q_re0=0.99  q_v1=0.008  longvl=17 m/s  cz=5e5 N/m  model_resistance=0  resistance_model=1  coeff=0.015  p_tire=250e3 Pa  alpha=-0.003  beta=0.97  coeff_a=84e-4  coeff_b=6.2e-4 s/m  coeff_c=1.6e-4 s^2/m^2  p_tire0=240e3 Pa  fz0_resistance=4000 N  vH0=16 m/s  q_Sy=[.0082, 0, .0014, .001, 0, 0, 1.08, -.5]  v_thr=1e-3 m/s  enable_scaling_coefficients=false  lfzO=1  lcx=1  lmux=1  lex=1  lkx=1  lhx=1  lvx=1  lmy=1  model_compliance=0  stiffness=1e+6 N/m  damping=1000 N/(m/s)  model_inertia=1  inertia=1e-2 kg*m^2  initial_velocity=0 rpm  vxlow=0.1 m/s  v_tr_thr=0.01 m/s  kpumin=-1.5  kpumax=1.5
  Vehicle Body : sdl_lib/Tires & Vehicles/Vehicle Body  mass=1200 kg  n_w=2  x_f=1.4 m  x_r=1.6 m  y_c=0.5 m  mass_var=simscape.enum.onoff.off  g=9.81 m/s^2  liftoff_warning=0  area=3 m^2  Cd_var=false  Cd=0.4  rho=1.18 kg/m^3  model_pitch=0  inertia=4000 kg*m^2  suspension_model=1  k_f=1e4 N/m  b_f=1e4 N/(m/s)  k_r=1e4 N/m  b_r=1e4 N/(m/s)  k_f_TLU=[-2000, -1000, 0, 1000, 2000] N  x_f_TLU=[-.4, -.2, 0, .2, .4] m  b_f_TLU=[-200, -100, 0, 100, 200] N  v_f_TLU=[-4, -2, 0, 2, 4] m/s  k_r_TLU=[-2000, -1000, 0, 1000, 2000] N  x_r_TLU=[-.4, -.2, 0, .2, .4] m  b_r_TLU=[-200, -100, 0, 100, 200] N  v_r_TLU=[-4, -2, 0, 2, 4] m/s  interp_method=simscape.enum.interpolation.linear  extrap_method=simscape.enum.extrapolation.linear  model_hardstop=0  upper_bound_f=.25 m  lower_bound_f=-.25 m  stop_k_f=1e6 N/m  stop_b_f=150 N/(m/s)  upper_bound_r=.25 m  lower_bound_r=-.25 m  stop_k_r=1e6 N/m  stop_b_r=150 N/(m/s)  initial_pitch=0 rad  initial_pitch_rate=0 rad/s  v_specify=off  v_priority=High  v=0 m/s  v_nominal_specify=off  v_nominal_value=1  v_nominal_unit=m/s
      settings: InternalSimscapePortConfiguration="{\"Bottom\":[{\"id\":\"NR\",\"label\":\"NR\",\"type\":\"output\"},{\"id\":\"NF\",\"label\":\"NF\",\"type\":\"output\"},{\"id\":\"beta\",\"label\":\"beta\",\"type\":\"input\"}],\"Left\":[{\"id\":\"H\",\"label\":\"H\",\"type\":\"foundation.mechanical.translational.translational\"}],\"Right\":[],\"Top\":[{\"id\":\"V\",\"label\":\"V\",\"type\":\"output\"},{\"id\":\"wind\",\"label\":\"W\",\"type\":\"input\"}]}"
  Wind Velocity : fl_lib/Physical Signals/Sources/PS Constant  constant=5
  A : PMIOPort  Side=Left
  v : Outport  VectorParamsAs1DForOutWhenUnconnected=off
  wires:
  PS-Simulink Converter3/1 -> v/1  "Velocity"
  PS-Simulink Converter1/1 -> Tire Slip/1  "Slip"
  Gain/1 -> Simulink-PS Converter/1
  Br/1 -> Gain/1
  Inclination/1 -> Simulink-PS Converter1/1
  connections:
  Wind Velocity/RConn1 -- Vehicle Body/LConn3
  PS-Simulink Converter3/LConn1 -- Vehicle Body/LConn2
  Vehicle Body/LConn1 -- Tire Left/RConn2 -- Tire Right/RConn2
  Vehicle Body/RConn1 -- Tire Right/LConn1 -- Tire Left/LConn1
  A/RConn1 -- Double-Shoe Brake/LConn2 -- Tire Right/LConn2 -- Tire Left/LConn2
  Tire Left/RConn1 -- PS-Simulink Converter1/LConn1
  Simulink-PS Converter/RConn1 -- Double-Shoe Brake/LConn1
  Simulink-PS Converter1/RConn1 -- Vehicle Body/RConn3

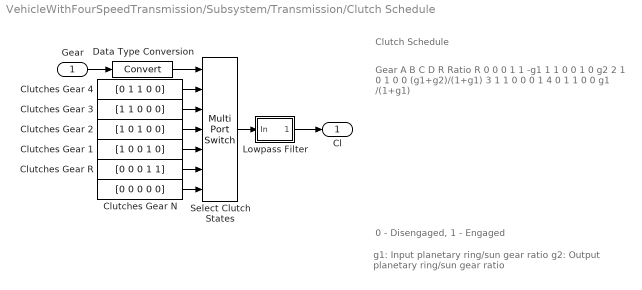
== system VehicleWithFourSpeedTransmission/Subsystem/Transmission/Clutch Schedule ==
  note: Gear
      | A
      | B
      | C
      | D
      | R
      | Ratio
      |
      | R
      | 0
      | 0
      | 0
      | 1
      | 1
      | -g1
      |
      | 1
      | 1
      | 0
      | 0
      | 1
      | 0
      | g2
      |
      | 2
      | 1
      | 0
      | 1
      | 0
      | 0
      | (g1+g2)/(1+g1)
      |
      | 3
      | 1
      | 1
      | 0
      | 0
      | 0
      | 1
      |
      | 4
      | 0
      | 1
      | 1
      | 0
      | 0
      | g1 /(1+g1)
  note: g1: Input planetary ring/sun gear ratio
      | g2: Output planetary ring/sun gear ratio
  note: 0 - Disengaged, 1 - Engaged
  note: Clutch Schedule
  Gear : Inport
  Clutches Gear 1 : Constant  Value=[1 0 0 1 0]  SampleTime=0
  Clutches Gear 2 : Constant  Value=[1 0 1 0 0]  SampleTime=0
  Clutches Gear 3 : Constant  Value=[1 1 0 0 0]  SampleTime=0
  Clutches Gear 4 : Constant  Value=[0 1 1 0 0]  SampleTime=0
  Clutches Gear N : Constant  Value=[0 0 0 0 0]  SampleTime=0
  Clutches Gear R : Constant  Value=[0 0 0 1 1]  SampleTime=0
  Data Type Conversion : DataTypeConversion  SaturateOnIntegerOverflow=off  RndMeth=Floor
  Lowpass Filter : Subsystem  mask(First-order lag supporting vector signals){b=0.05, x_initial=[0 0 0 0 0]}
      mask prompts: b "Filter time constant"; x_initial "Initial output"
      mask help: Models a lag of the form 1/(b*s+1) where s is the Laplace operator.
  Select Clutch States : MultiPortSwitch  DataPortOrder=Specify indices  DataPortIndices={4,3,2,1,-1,0}  DiagnosticForDefault=None  SaturateOnIntegerOverflow=off  InputSameDT=off
  Cl : Outport  VectorParamsAs1DForOutWhenUnconnected=off
  wires:
  Clutches Gear 4/1 -> Select Clutch States/2
  Clutches Gear 2/1 -> Select Clutch States/4
  Clutches Gear 1/1 -> Select Clutch States/5
  Clutches Gear N/1 -> Select Clutch States/7
  Clutches Gear R/1 -> Select Clutch States/6
  Clutches Gear 3/1 -> Select Clutch States/3
  Select Clutch States/1 -> Lowpass Filter/1(In)
  Data Type Conversion/1 -> Select Clutch States/1
  Lowpass Filter/1(Out) -> Cl/1
  Gear/1 -> Data Type Conversion/1

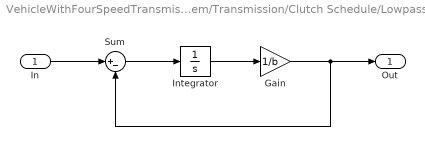
== system VehicleWithFourSpeedTransmission/Subsystem/Transmission/Clutch Schedule/Lowpass Filter ==
  In : Inport
  Gain : Gain  Gain=1/b
  Integrator : Integrator  InitialCondition=x_initial*b
  Sum : Sum  Inputs=|+-  InputSameDT=on  SaturateOnIntegerOverflow=on  OutDataTypeStr=Inherit: Same as first input
  Out : Outport  VectorParamsAs1DForOutWhenUnconnected=off
  wires:
  Sum/1 -> Integrator/1
  In/1 -> Sum/1
  Integrator/1 -> Gain/1
  Gain/1 -> Sum/2, Out/1

== stateflow chart VehicleWithFourSpeedTransmission/Subsystem/Shift Logic ==
  settings: updateMethod=DISCRETE  sampleTime=0.04
  state gear_state [parallel]
    settings: executionOrder=1
    state first
      entry:
      Gear = 1;
    state second
      entry:
      Gear = 2;
    state third
      entry:
      Gear = 3;
    state fourth
      entry:
      Gear = 4;
    (default) -> first
    second -> third [order 1] : UP
    first -> second : UP
    third -> fourth [order 1] : UP
    third -> second [order 2] : DOWN
    second -> first [order 2] : DOWN
    fourth -> third : DOWN
  state selection_state [parallel]
    during:
    [down_th, up_th] = ComputeThreshold(Gear,Throttle);
    settings: executionOrder=2
    state steady_state
    state upshifting
    state downshifting
    (default) -> steady_state
    steady_state -> upshifting [order 1] : [VehicleSpeed > up_th]
    steady_state -> downshifting [order 2] : [VehicleSpeed < down_th]
    downshifting -> steady_state [order 2] : [VehicleSpeed > down_th]
    downshifting -> steady_state [order 1] : after(TWAIT,tick)
        | [VehicleSpeed <= down_th]
        | {gear_state.DOWN;}
    upshifting -> steady_state [order 1] : after(TWAIT,tick)
        | [VehicleSpeed >= up_th]
        | {gear_state.UP;}
    upshifting -> steady_state [order 2] : [VehicleSpeed < up_th]
  state [down_th,up_th] = ComputeThreshold(Gear,Throttle) [function]
  data: Gear function_input; Throttle function_input; down_th function_output; up_th function_output; VehicleSpeed input double; Throttle input double; Gear output double [1..4]; TWAIT parameter double; down_th local double; up_th local double
  events: DOWN local EITHER_EDGE_EVENT; UP local EITHER_EDGE_EVENT
